simulink model "referenced"  (R2020a)
settings: Solver=FixedStepAuto  StartTime=0.0  StopTime=10.0  FixedStep=0.2  RelTol=1e-3
settings Model: Creator=Admin  LastModifiedBy=Admin
settings DataIOCC: SaveOutput=off  SaveTime=off

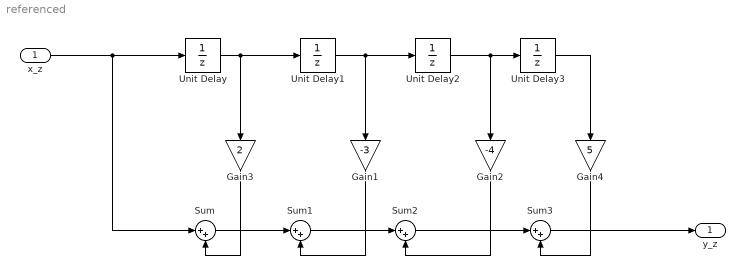
== system referenced ==
  x_z : Inport  OutDataTypeStr=double  PortDimensions=1  SampleTime=[0.20000000000000001,0]
  Gain1 : Gain  Gain=-3
  Gain2 : Gain  Gain=-4
  Gain3 : Gain  Gain=2
  Gain4 : Gain  Gain=5
  Sum{,1..3} (4 alike) : Sum  Inputs=|++
  Unit Delay{,1..3} (4 alike) : UnitDelay  SampleTime=-1  HasFrameUpgradeWarning=on
  y_z : Outport  OutDataTypeStr=double  PortDimensions=1  SampleTime=[0.20000000000000001,0]
  wires:
  x_z/1 -> Sum/1, Unit Delay/1
  Unit Delay2/1 -> Unit Delay3/1, Gain2/1
  Sum3/1 -> y_z/1
  Unit Delay3/1 -> Gain4/1
  Unit Delay1/1 -> Unit Delay2/1, Gain1/1
  Unit Delay/1 -> Unit Delay1/1, Gain3/1
  Gain3/1 -> Sum/2
  Sum/1 -> Sum1/1
  Gain1/1 -> Sum1/2
  Sum1/1 -> Sum2/1
  Gain2/1 -> Sum2/2
  Sum2/1 -> Sum3/1
  Gain4/1 -> Sum3/2
